simulink model "GNC_integrated"  (R2023a)
settings: Solver=VariableStepAuto  StartTime=0.0  StopTime=200  RelTol=1e-3
undefined symbols (not defined in the file or in its folder): param
libraries: eeGeneralControl x12, simulink_extras x6, uavalgslib x3, simulink x2, SignalEditorBlockLib x1, sharedTrackingLibrary x1
settings Model: Creator=timme  LastModifiedBy=jipva

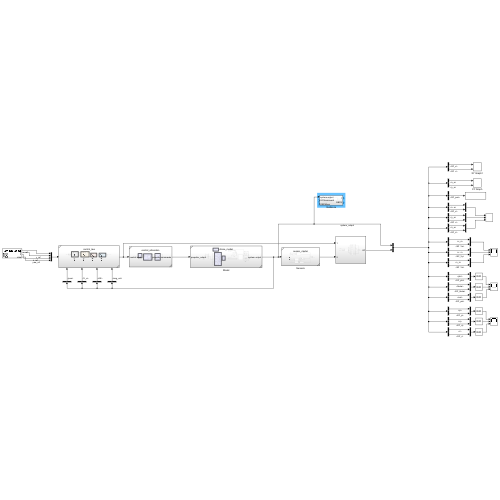
[thumbnail: Simulink's stored preview of the top-level diagram]
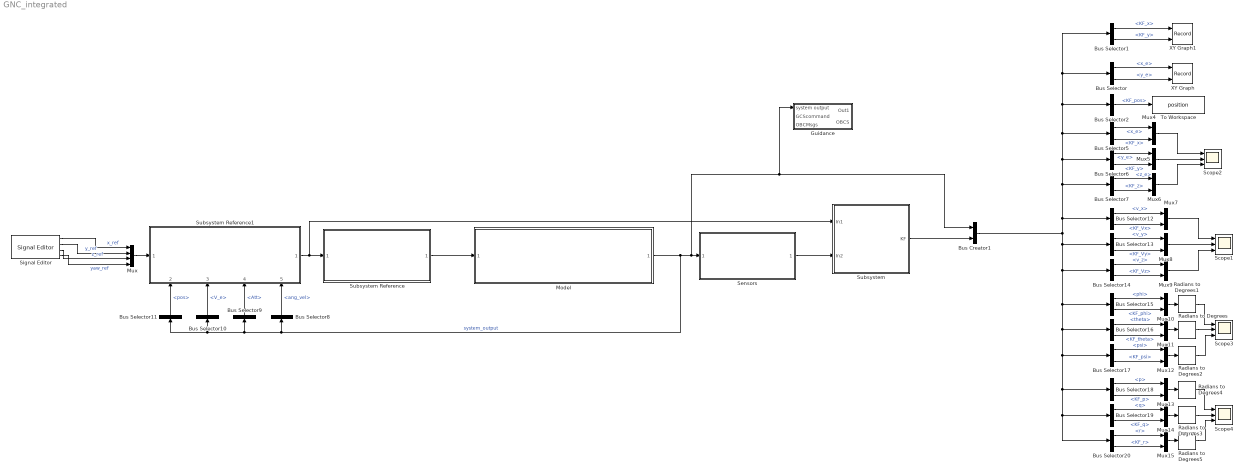
== system GNC_integrated ==
  Bus Creator1 : BusCreator  Inputs=2
  Bus Selector : BusSelector  OutputSignals=system_output.pos.x_e,system_output.pos.y_e
  Bus Selector1 : BusSelector  OutputSignals=KF.KF_pos.KF_x,KF.KF_pos.KF_y
  Bus Selector10 : BusSelector  OutputSignals=V_e
  Bus Selector11 : BusSelector  OutputSignals=pos
  Bus Selector12 : BusSelector  OutputSignals=system_output.V_e.v_x,KF.KF_vel.KF_Vx
  Bus Selector13 : BusSelector  OutputSignals=system_output.V_e.v_y,KF.KF_vel.KF_Vy
  Bus Selector14 : BusSelector  OutputSignals=system_output.V_e.v_z,KF.KF_vel.KF_Vz
  Bus Selector15 : BusSelector  OutputSignals=system_output.Att.phi,KF.KF_att.KF_phi
  Bus Selector16 : BusSelector  OutputSignals=system_output.Att.theta,KF.KF_att.KF_theta
  Bus Selector17 : BusSelector  OutputSignals=system_output.Att.psi,KF.KF_att.KF_psi
  Bus Selector18 : BusSelector  OutputSignals=system_output.ang_vel.p,KF.KF_omega.KF_p
  Bus Selector19 : BusSelector  OutputSignals=system_output.ang_vel.q,KF.KF_omega.KF_q
  Bus Selector2 : BusSelector  OutputSignals=KF.KF_pos
  Bus Selector20 : BusSelector  OutputSignals=system_output.ang_vel.r,KF.KF_omega.KF_r
  Bus Selector5 : BusSelector  OutputSignals=system_output.pos.x_e,KF.KF_pos.KF_x
  Bus Selector6 : BusSelector  OutputSignals=system_output.pos.y_e,KF.KF_pos.KF_y
  Bus Selector7 : BusSelector  OutputSignals=system_output.pos.z_e,KF.KF_pos.KF_z
  Bus Selector8 : BusSelector  OutputSignals=ang_vel
  Bus Selector9 : BusSelector  OutputSignals=Att
  Guidance : Subsystem
  Model : Subsystem  ReferencedSubsystem=drone_model
  Mux : Mux
  Mux{4..15} (12 alike) : Mux  Inputs=2
  Radians to Degrees{,1..5} (6 alike) : simulink_extras/Transformations/Radians to Degrees
  Scope{1..4} (4 alike) : Scope  NumInputPorts=3
  Sensors : Subsystem  ReferencedSubsystem=sensor_model
  Signal Editor : SignalEditorBlockLib/Signal Editor  FileName=C:\Users\jipva\MATLAB\Projects\drone\Detailed design phase\guidance\full_system_reference.mat  ActiveScenario=StandardScenario  ActiveSignal=yaw  IsBus=off  OutputBusObjectStr=Bus: BusObject  SampleTime=param.dt  ZeroCross=off  OutputAfterFinalValue=Setting to zero  Unit=inherit  PreserveSignalName=on  ApplySigPropsToAllScenarios=on
  Subsystem : Subsystem
  Subsystem Reference : Subsystem  ReferencedSubsystem=control_allocation
  Subsystem Reference1 : Subsystem  ReferencedSubsystem=control_law
      settings: PortSchema="{\"entries\":[{\"content\":{\"sides\":[{\"content\":{\"connectorIds\":[\"In1\"]},\"type\":\"ConnectorPlacement.EquallySpacedRectSide\",\"uuid\":\"cbb659e7-d19a-4e68-9ae7-e5e39426296b\"},{\"content\":{\"connectorIds\":[\"Out1\"],\"side\":\"RIGHT\"},\"type\":\"ConnectorPlacement.EquallySpacedRectSide\",\"uuid\":\"c9f08a4e-80d9-41bf-93e6-4cfd11b32426\"},{\"content\":{\"side\":\"TOP\"},\"type\":\"ConnectorPlacement.EquallySpacedRectSide\",\"uuid\":\"8eafc22d-128e-4ca7-9eba-2c3fd299252c\"},{\"content\":{\"connectorIds\":[\"In2\",\"In3\",\"In4\",\"In5\"],\"side\":\"BOTTOM\"},\"type\":\"ConnectorPlacement.EquallySpacedRectSide\",\"uuid\":\"abe1dc09-e6b8-433e-beaf-ba54ebcb4b47\"}]},\"type\":\"ConnectorPlacement.EquallySpacedConnector\",\"uuid\":\"085ffc95-65e8-4235-be8d-72c324b16b8b\"}],\"packageUris\":[\"http://schema.mathworks.com/mf0/Connector/R2020b\"],\"version\":\"1.0\"}"
  To Workspace : ToWorkspace  VariableName=position  SaveFormat=Timeseries  SampleTime=param.dt
  XY Graph : Record  FileSettingsInternal="{\"entries\":[{\"content\":{\"excelSettings\":{\"content\":{},\"type\":\"Streamout.ExcelSettings\"}},\"type\":\"Streamout.FileSettingStorage\",\"uuid\":\"\"}],\"packageUris\":[\"http:\\/\\/schema.mathworks.com\\/mf0\\/streamout_blocks\\/R2020a\"],\"version\":\"1.0\"}"  Layout=[1 1]  SignalsInternal="{\"entries\":[{\"content\":{\"signals\":[{\"content\":{\"blockPath\":[],\"dimensions\":[1],\"domain\":\"\",\"lineColor\":\"#a2142f\",\"plots\":[1],\"port\":1,\"signalID\":34,\"signalName\":\"<x_e>\"},\"type\":\"RecordBlkView.Signal\",\"uuid\":\"\"},{\"content\":{\"blockPath\":[],\"dimensions\":[1],\"domain\":\"\",\"lineColor\":\"#139fff\",\"plots\":[1],\"port\":2,\"signalID\":37,\"signalName\":\"<y_e>\"},\"type\":\"RecordBlkView.Signal\",\"uuid\":\"\"}]},\"type\":\"RecordBlkView.InputSignals\",\"uuid\":\"\"}],\"packageUris\":[\"http:\\/\\/schema.mathworks.com\\/mf0\\/streamout_blocks\\/R2020a\"],\"version\":\"1.0\"}"  VisualizationBindings="{\"xyplotplugin\":{\"info\":[{\"series\":[{\"bindingParametersList\":[{\"parameter\":\"X-Axis\",\"signalID\":34,\"signalName\":\"<x_e>\"},{\"parameter\":\"Y-Axis\",\"signalID\":37,\"signalName\":\"<y_e>\"}],\"seriesID\":47186}],\"subplotID\":1}]}}"  CompatibilityTag=XY
  XY Graph1 : Record  FileSettingsInternal="{\"entries\":[{\"content\":{\"excelSettings\":{\"content\":{},\"type\":\"Streamout.ExcelSettings\"}},\"type\":\"Streamout.FileSettingStorage\",\"uuid\":\"\"}],\"packageUris\":[\"http:\\/\\/schema.mathworks.com\\/mf0\\/streamout_blocks\\/R2020a\"],\"version\":\"1.0\"}"  Layout=[1 1]  SignalsInternal="{\"entries\":[{\"content\":{\"signals\":[{\"content\":{\"blockPath\":[],\"dimensions\":[1],\"domain\":\"\",\"lineColor\":\"#a2142f\",\"plots\":[1],\"port\":1,\"signalID\":26,\"signalName\":\"Second-Order Filter3\"},\"type\":\"RecordBlkView.Signal\",\"uuid\":\"\"},{\"content\":{\"blockPath\":[],\"dimensions\":[1],\"domain\":\"\",\"lineColor\":\"#139fff\",\"plots\":[1],\"port\":2,\"signalID\":29,\"signalName\":\"Second-Order Filter4\"},\"type\":\"RecordBlkView.Signal\",\"uuid\":\"\"}]},\"type\":\"RecordBlkView.InputSignals\",\"uuid\":\"\"}],\"packageUris\":[\"http:\\/\\/schema.mathworks.com\\/mf0\\/streamout_blocks\\/R2020a\"],\"version\":\"1.0\"}"  VisualizationBindings="{\"xyplotplugin\":{\"info\":[{\"series\":[{\"bindingParametersList\":[{\"parameter\":\"X-Axis\",\"signalID\":26,\"signalName\":\"Second-Order Filter3\"},{\"parameter\":\"Y-Axis\",\"signalID\":29,\"signalName\":\"Second-Order Filter4\"}],\"seriesID\":35333}],\"subplotID\":1}]}}"  CompatibilityTag=XY
  wires:
  Model/1 -> Guidance/1(system output), Bus Creator1/1, Sensors/1, Bus Selector11/1, Bus Selector10/1, Bus Selector9/1, Bus Selector8/1  "system_output"
  Subsystem Reference1/1 -> Subsystem/1(In1), Subsystem Reference/1
  Bus Selector5/1 -> Mux4/1  "<x_e>"
  Bus Selector5/2 -> Mux4/2  "<KF_x>"
  Bus Selector6/1 -> Mux5/1  "<y_e>"
  Bus Selector6/2 -> Mux5/2  "<KF_y>"
  Bus Selector7/2 -> Mux6/2  "<KF_z>"
  Bus Selector7/1 -> Mux6/1  "<z_e>"
  Bus Selector8/1 -> Subsystem Reference1/5  "<ang_vel>"
  Bus Selector9/1 -> Subsystem Reference1/4  "<Att>"
  Bus Selector10/1 -> Subsystem Reference1/3  "<V_e>"
  Bus Selector11/1 -> Subsystem Reference1/2  "<pos>"
  Bus Selector12/2 -> Mux7/2  "<KF_Vx>"
  Bus Selector12/1 -> Mux7/1  "<v_x>"
  Bus Selector13/1 -> Mux8/1  "<v_y>"
  Bus Selector14/2 -> Mux9/2  "<KF_Vz>"
  Bus Selector14/1 -> Mux9/1  "<v_z>"
  Bus Selector13/2 -> Mux8/2  "<KF_Vy>"
  Bus Selector16/2 -> Mux11/2  "<KF_theta>"
  Mux12/1 -> Radians to Degrees2/1
  Mux11/1 -> Radians to Degrees/1
  Bus Selector17/2 -> Mux12/2  "<KF_psi>"
  Bus Selector17/1 -> Mux12/1  "<psi>"
  Bus Selector15/2 -> Mux10/2  "<KF_phi>"
  Mux10/1 -> Radians to Degrees1/1
  Bus Selector15/1 -> Mux10/1  "<phi>"
  Bus Selector16/1 -> Mux11/1  "<theta>"
  Bus Selector19/2 -> Mux14/2  "<KF_q>"
  Bus Selector18/2 -> Mux13/2  "<KF_p>"
  Mux13/1 -> Radians to Degrees4/1
  Bus Selector20/1 -> Mux15/1  "<r>"
  Bus Selector18/1 -> Mux13/1  "<p>"
  Mux15/1 -> Radians to Degrees5/1
  Bus Selector20/2 -> Mux15/2  "<KF_r>"
  Mux14/1 -> Radians to Degrees3/1
  Bus Selector19/1 -> Mux14/1  "<q>"
  Signal Editor/2 -> Mux/2  "y_ref"
  Signal Editor/1 -> Mux/1  "x_ref"
  Signal Editor/3 -> Mux/3  "z_ref"
  Signal Editor/4 -> Mux/4  "yaw_ref"
  Mux/1 -> Subsystem Reference1/1
  Subsystem Reference/1 -> Model/1
  Bus Selector/1 -> XY Graph/1  "<x_e>"
  Bus Selector/2 -> XY Graph/2  "<y_e>"
  Bus Creator1/1 -> Bus Selector13/1, Bus Selector14/1, Bus Selector20/1, Bus Selector19/1, Bus Selector18/1, Bus Selector17/1, Bus Selector16/1, Bus Selector15/1, Bus Selector12/1, Bus Selector7/1, Bus Selector6/1, Bus Selector2/1, Bus Selector1/1, Bus Selector/1, Bus Selector5/1
  Mux5/1 -> Scope2/2
  Mux4/1 -> Scope2/1
  Mux6/1 -> Scope2/3
  Mux8/1 -> Scope1/2
  Mux9/1 -> Scope1/3
  Mux7/1 -> Scope1/1
  Radians to Degrees2/1 -> Scope3/3
  Radians to Degrees1/1 -> Scope3/1
  Radians to Degrees/1 -> Scope3/2
  Radians to Degrees5/1 -> Scope4/3
  Radians to Degrees4/1 -> Scope4/1
  Radians to Degrees3/1 -> Scope4/2
  Bus Selector1/1 -> XY Graph1/1  "<KF_x>"
  Bus Selector1/2 -> XY Graph1/2  "<KF_y>"
  Sensors/1 -> Subsystem/2(In2)
  Subsystem/1(KF) -> Bus Creator1/2
  Bus Selector2/1 -> To Workspace/1  "<KF_pos>"

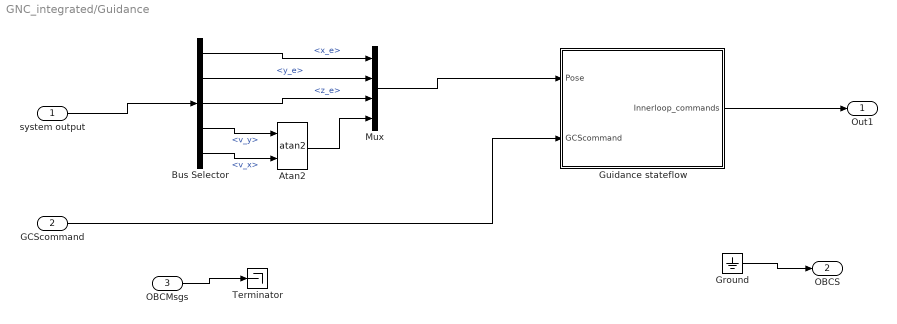
== system GNC_integrated/Guidance ==
  system output : Inport
  GCScommand : Inport  Port=2
  OBCMsgs : Inport  Port=3
  Atan2 : Trigonometry  Operator=atan2
  Bus Selector : BusSelector  OutputSignals=pos.x_e,pos.y_e,pos.z_e,V_e.v_y,V_e.v_x
  Ground : Ground
  Guidance stateflow : Subsystem
  Mux : Mux
  Terminator : Terminator
  Out1 : Outport
  OBCS : Outport  Port=2
  wires:
  system output/1 -> Bus Selector/1
  Bus Selector/4 -> Atan2/1  "<v_y>"
  Bus Selector/5 -> Atan2/2  "<v_x>"
  Bus Selector/3 -> Mux/3  "<z_e>"
  Bus Selector/2 -> Mux/2  "<y_e>"
  Bus Selector/1 -> Mux/1  "<x_e>"
  Atan2/1 -> Mux/4
  Mux/1 -> Guidance stateflow/1(Pose)
  GCScommand/1 -> Guidance stateflow/2(GCScommand)
  OBCMsgs/1 -> Terminator/1
  Guidance stateflow/1(Innerloop_commands) -> Out1/1
  Ground/1 -> OBCS/1

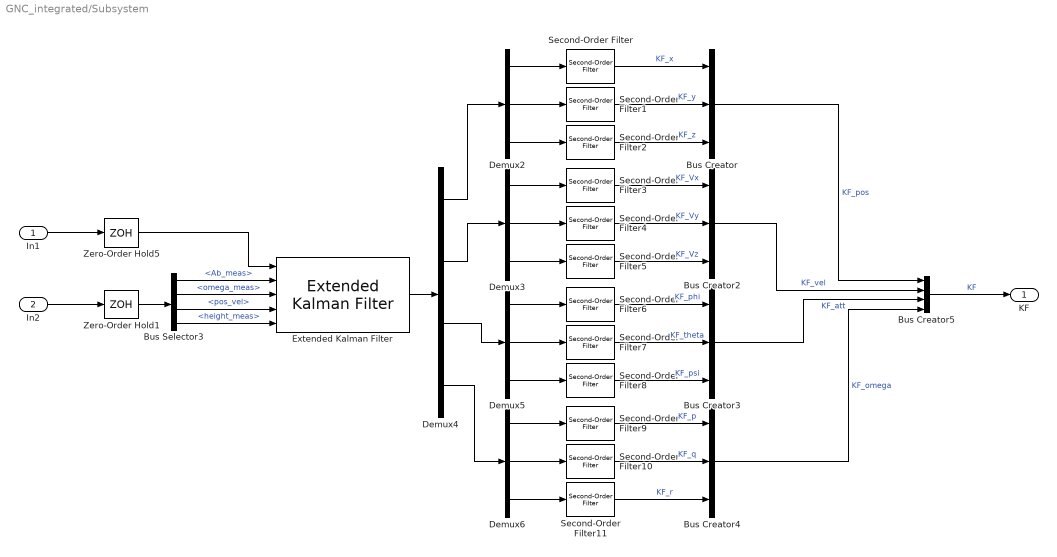
== system GNC_integrated/Subsystem ==
  In1 : Inport
  In2 : Inport  Port=2
  Bus Creator{,2..4} (4 alike) : BusCreator  Inputs=3
  Bus Creator5 : BusCreator  Inputs=4
  Bus Selector3 : BusSelector  OutputSignals=Ab_meas,omega_meas,pos_vel,height_meas
  Demux{2..3,5..6} (4 alike) : Demux  Outputs=3
  Demux4 : Demux
  Extended Kalman Filter : sharedTrackingLibrary/Extended Kalman Filter  StateTransitionFcn=stateTransition  HasStateTransitionJacobianFcn=off  HasAdditiveProcessNoise=Additive  ProcessNoise=10  HasTimeVaryingProcessNoise=off  HasStateTransitionFcnExtraArgument=1  InitialState=zeros(12,1)  InitialStateCovariance=zeros(12)  MeasurementFcn1=accelerometer_model  HasMeasurementJacobianFcn1=off  HasMeasurementEnablePort1=off  HasAdditiveMeasurementNoise1=Additive  MeasurementNoise1=diag([100 100 100])  HasTimeVaryingMeasurementNoise1=off  HasMeasurementFcnExtraArgument1=0  HasMeasurementWrapping1=off  MeasurementFcn2=gyrometer_model  HasMeasurementJacobianFcn2=off  HasMeasurementEnablePort2=off  HasAdditiveMeasurementNoise2=Additive  MeasurementNoise2=eye(3)  HasTimeVaryingMeasurementNoise2=off  HasMeasurementFcnExtraArgument2=0  HasMeasurementWrapping2=off  MeasurementFcn3=GPS_model  HasMeasurementJacobianFcn3=off  HasMeasurementEnablePort3=off  HasAdditiveMeasurementNoise3=Additive  MeasurementNoise3=diag([10 10 100 0.1 0.1 0.1])  HasTimeVaryingMeasurementNoise3=off  HasMeasurementFcnExtraArgument3=0  HasMeasurementWrapping3=off  MeasurementFcn4=Barometer_model  HasMeasurementJacobianFcn4=off  HasMeasurementEnablePort4=off  HasAdditiveMeasurementNoise4=Additive  MeasurementNoise4=0.01  HasTimeVaryingMeasurementNoise4=off  HasMeasurementFcnExtraArgument4=0  HasMeasurementWrapping4=off  MeasurementFcn5=myMeasurementFcn  HasMeasurementJacobianFcn5=off  HasMeasurementEnablePort5=off  HasAdditiveMeasurementNoise5=Additive  MeasurementNoise5=1  HasTimeVaryingMeasurementNoise5=off  HasMeasurementFcnExtraArgument5=0  HasMeasurementWrapping5=off  EnableMultirate=off  StateTransitionFcnSampleTime=1  MeasurementFcn1SampleTime=1  MeasurementFcn2SampleTime=1  MeasurementFcn3SampleTime=1  MeasurementFcn4SampleTime=1  MeasurementFcn5SampleTime=1  UseCurrentEstimator=on  OutputStateCovariance=off  DataType=double  SampleTime=0.01  NumberOfMeasurements=4
  Second-Order Filter{,1..11} (12 alike) : eeGeneralControl/Second-Order Filter  FilterType=Low-pass  fn=10  Zeta=0.707  Ts=param.dt  A0=0  Ph0=0  f0=0  b0=0
      settings: LibrarySourceBlock=ee_sl_lib/General Control/Second-Order Filter
  Zero-Order Hold1 : ZeroOrderHold  SampleTime=param.dt
  Zero-Order Hold5 : ZeroOrderHold  SampleTime=param.dt
  KF : Outport
  wires:
  Demux5/2 -> Second-Order Filter7/1
  Bus Selector3/2 -> Extended Kalman Filter/3  "<omega_meas>"
  Demux6/1 -> Second-Order Filter9/1
  Bus Selector3/3 -> Extended Kalman Filter/4  "<pos_vel>"
  Demux2/3 -> Second-Order Filter2/1
  Zero-Order Hold5/1 -> Extended Kalman Filter/1
  Demux3/1 -> Second-Order Filter3/1
  Zero-Order Hold1/1 -> Bus Selector3/1
  Demux6/2 -> Second-Order Filter10/1
  Demux6/3 -> Second-Order Filter11/1
  Demux5/3 -> Second-Order Filter8/1
  Bus Creator2/1 -> Bus Creator5/2  "KF_vel"
  Bus Creator/1 -> Bus Creator5/1  "KF_pos"
  Demux4/2 -> Demux3/1
  Demux3/3 -> Second-Order Filter5/1
  Demux2/1 -> Second-Order Filter/1
  Bus Creator4/1 -> Bus Creator5/4  "KF_omega"
  Demux4/1 -> Demux2/1
  Demux5/1 -> Second-Order Filter6/1
  Bus Selector3/1 -> Extended Kalman Filter/2  "<Ab_meas>"
  Demux3/2 -> Second-Order Filter4/1
  Bus Selector3/4 -> Extended Kalman Filter/5  "<height_meas>"
  Bus Creator3/1 -> Bus Creator5/3  "KF_att"
  Demux4/4 -> Demux6/1
  In2/1 -> Zero-Order Hold1/1
  Second-Order Filter1/1 -> Bus Creator/2  "KF_y"
  Extended Kalman Filter/1 -> Demux4/1
  Demux4/3 -> Demux5/1
  Bus Creator5/1 -> KF/1  "KF"
  In1/1 -> Zero-Order Hold5/1
  Second-Order Filter/1 -> Bus Creator/1  "KF_x"
  Demux2/2 -> Second-Order Filter1/1
  Second-Order Filter2/1 -> Bus Creator/3  "KF_z"
  Second-Order Filter3/1 -> Bus Creator2/1  "KF_Vx"
  Second-Order Filter4/1 -> Bus Creator2/2  "KF_Vy"
  Second-Order Filter5/1 -> Bus Creator2/3  "KF_Vz"
  Second-Order Filter6/1 -> Bus Creator3/1  "KF_phi"
  Second-Order Filter7/1 -> Bus Creator3/2  "KF_theta"
  Second-Order Filter8/1 -> Bus Creator3/3  "KF_psi"
  Second-Order Filter9/1 -> Bus Creator4/1  "KF_p"
  Second-Order Filter10/1 -> Bus Creator4/2  "KF_q"
  Second-Order Filter11/1 -> Bus Creator4/3  "KF_r"

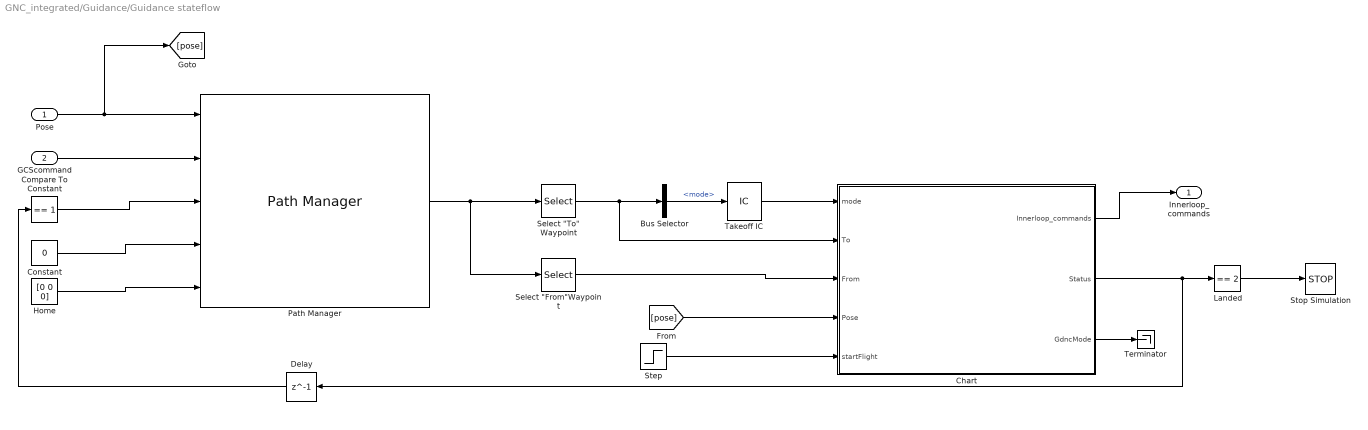
== system GNC_integrated/Guidance/Guidance stateflow ==
  Pose : Inport
  GCScommand : Inport  Port=2
  Bus Selector : BusSelector  OutputSignals=mode
  Chart : Stateflow chart  TreatAsAtomicUnit=on
      settings: PortSchema="{\"entries\":[{\"content\":{\"sides\":[{\"content\":{\"connectorIds\":[\"In1\",\"In3\",\"In4\",\"In2\",\"In5\"]},\"type\":\"ConnectorPlacement.EquallySpacedRectSide\",\"uuid\":\"d234d877-22d9-4518-b5ba-a604db0bf90b\"},{\"content\":{\"connectorIds\":[\"Out1\",\"Out2\",\"Out3\"],\"side\":\"RIGHT\"},\"type\":\"ConnectorPlacement.EquallySpacedRectSide\",\"uuid\":\"0dfe34a8-7c44-4a97-9042-ef916a7aa529\"},{\"content\":{\"side\":\"TOP\"},\"type\":\"ConnectorPlacement.EquallySpacedRectSide\",\"uuid\":\"69e1da7c-b0a2-43d5-a7f5-1531e368ea9d\"}]},\"type\":\"ConnectorPlacement.EquallySpacedConnector\",\"uuid\":\"b60a6dee-5aca-438c-8d1f-1665cdae5849\"}],\"packageUris\":[\"http://schema.mathworks.com/mf0/Connector/R2020b\"],\"version\":\"1.0\"}"
  Compare To Constant : simulink/Logic and Bit Operations/Compare To Constant  relop===  const=1  OutDataTypeStr=boolean
  Constant : Constant  Value=0
  Delay : Delay  DelayLength=1  InitialCondition=0
  Home : Constant  Value=[0 0 0]
  Landed : simulink/Logic and Bit Operations/Compare To Constant  relop===  const=2  OutDataTypeStr=boolean
  Path Manager : uavalgslib/Path Manager  UAVType=multirotor  LoiterRadius=25  dataType=double  inputBusName='UAVPathManagerBus'  SimulateUsing=Interpreted execution
  "Select \"From\"Waypoint" : Selector  InputPortWidth=2  IndexOptions=Index vector (dialog)  Indices=2  OutputSizes=1
  "Select \"To\" Waypoint" : Selector  InputPortWidth=2  IndexOptions=Index vector (dialog)  Indices=1  OutputSizes=1
  Step : Step  Time=0.5  SampleTime=0.02
  Stop Simulation : Stop
  Takeoff IC : InitialCondition
  Terminator : Terminator
  Innerloop_commands : Outport
  wires:
  Pose/1 -> [pose], Path Manager/1
  GCScommand/1 -> Path Manager/2
  Home/1 -> Path Manager/5
  Constant/1 -> Path Manager/4
  Path Manager/1 -> "Select \"From\"Waypoint"/1, "Select \"To\" Waypoint"/1
  "Select \"To\" Waypoint"/1 -> Chart/3(To), Bus Selector/1
  Bus Selector/1 -> Takeoff IC/1  "<mode>"
  "Select \"From\"Waypoint"/1 -> Chart/4(From)
  Delay/1 -> Compare To Constant/1
  Compare To Constant/1 -> Path Manager/3
  [pose] -> Chart/2(Pose)
  Chart/1(Innerloop_commands) -> Innerloop_commands/1
  Takeoff IC/1 -> Chart/1(mode)
  Step/1 -> Chart/5(startFlight)
  Chart/3(GdncMode) -> Terminator/1
  Chart/2(Status) -> Delay/1, Landed/1
  Landed/1 -> Stop Simulation/1

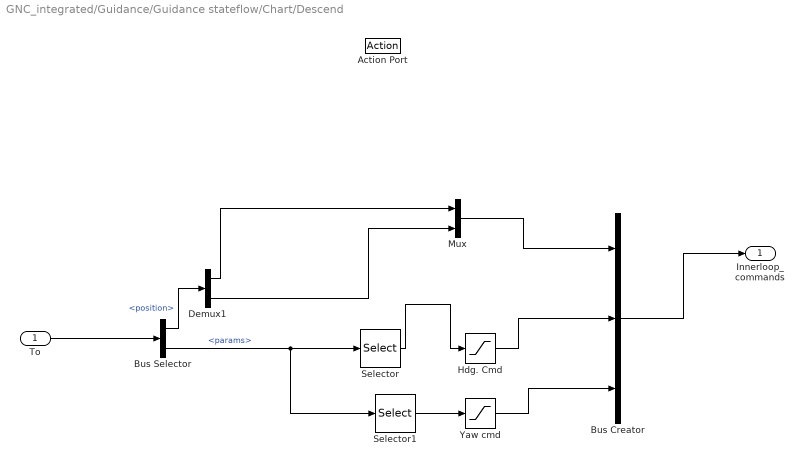
== system GNC_integrated/Guidance/Guidance stateflow/Chart/Descend ==
  To : Inport
  Action Port : ActionPort
      settings: CopyFcn=Stateflow.SLINSF.SimulinkMan.removeBlockPreDeleteFcn  PreDeleteFcn=Stateflow.SLINSF.SimulinkMan.unsafePredeleteFcn
  Bus Creator : BusCreator  Inputs=3
  Bus Selector : BusSelector  OutputSignals=position,params
  Demux1 : Demux  Outputs=2
  Hdg. Cmd : Saturate
  Mux : Mux  Inputs=2
  Selector : Selector  InputPortWidth=4  IndexOptions=Index vector (dialog)  Indices=4  OutputSizes=1
  Selector1 : Selector  InputPortWidth=4  IndexOptions=Index vector (dialog)  Indices=4  OutputSizes=1
  Yaw cmd : Saturate  UpperLimit=pi  LowerLimit=-pi
  Innerloop_commands : Outport
  wires:
  Bus Selector/1 -> Demux1/1  "<position>"
  Demux1/2 -> Mux/2
  Mux/1 -> Bus Creator/1
  Bus Selector/2 -> Selector1/1, Selector/1  "<params>"
  Selector1/1 -> Yaw cmd/1
  Demux1/1 -> Mux/1
  Hdg. Cmd/1 -> Bus Creator/2
  Selector/1 -> Hdg. Cmd/1
  Yaw cmd/1 -> Bus Creator/3
  Bus Creator/1 -> Innerloop_commands/1
  To/1 -> Bus Selector/1

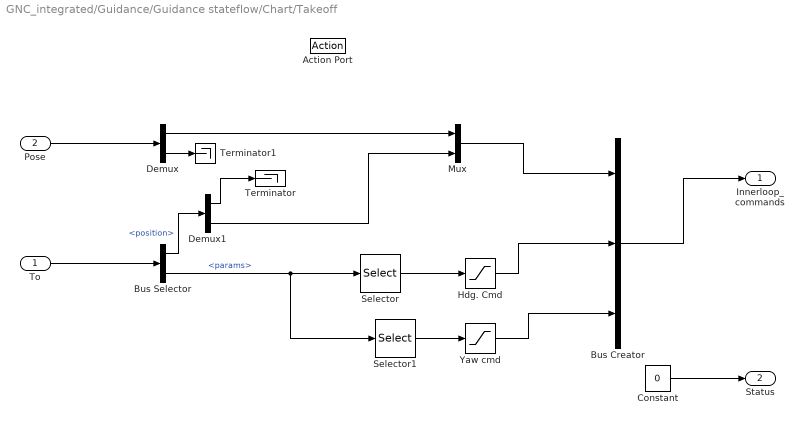
== system GNC_integrated/Guidance/Guidance stateflow/Chart/Takeoff ==
  To : Inport
  Pose : Inport  Port=2
  Action Port : ActionPort
      settings: CopyFcn=Stateflow.SLINSF.SimulinkMan.removeBlockPreDeleteFcn  PreDeleteFcn=Stateflow.SLINSF.SimulinkMan.unsafePredeleteFcn
  Bus Creator : BusCreator  Inputs=3
  Bus Selector : BusSelector  OutputSignals=position,params
  Constant : Constant  Value=0
  Demux : Demux  Outputs=2
  Demux1 : Demux  Outputs=2
  Hdg. Cmd : Saturate
  Mux : Mux  Inputs=2
  Selector : Selector  InputPortWidth=4  IndexOptions=Index vector (dialog)  Indices=4  OutputSizes=1
  Selector1 : Selector  InputPortWidth=4  IndexOptions=Index vector (dialog)  Indices=4  OutputSizes=1
  Terminator : Terminator
  Terminator1 : Terminator
  Yaw cmd : Saturate  UpperLimit=pi  LowerLimit=-pi
  Innerloop_commands : Outport
  Status : Outport  Port=2
  wires:
  Pose/1 -> Demux/1
  Demux/1 -> Mux/1
  Mux/1 -> Bus Creator/1
  To/1 -> Bus Selector/1
  Bus Selector/1 -> Demux1/1  "<position>"
  Demux1/1 -> Terminator/1
  Demux1/2 -> Mux/2
  Bus Selector/2 -> Selector1/1, Selector/1  "<params>"
  Bus Creator/1 -> Innerloop_commands/1
  Demux/2 -> Terminator1/1
  Hdg. Cmd/1 -> Bus Creator/2
  Selector1/1 -> Yaw cmd/1
  Selector/1 -> Hdg. Cmd/1
  Yaw cmd/1 -> Bus Creator/3
  Constant/1 -> Status/1

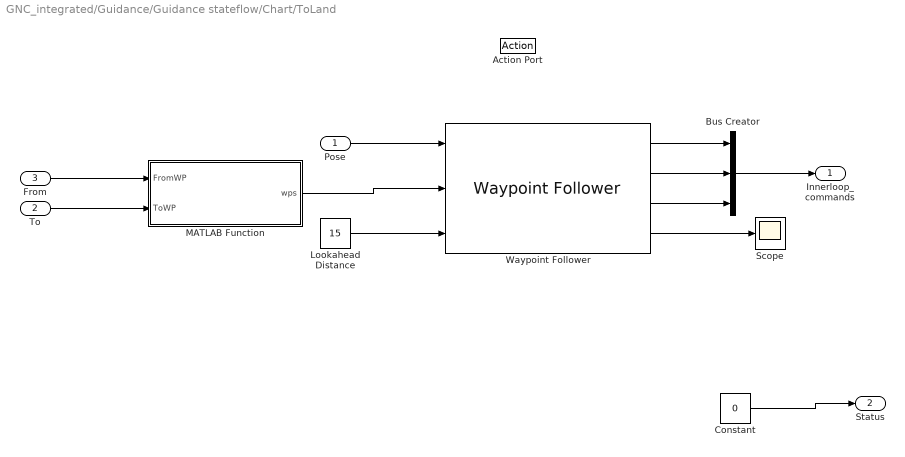
== system GNC_integrated/Guidance/Guidance stateflow/Chart/ToLand ==
  Pose : Inport
  To : Inport  Port=2
  From : Inport  Port=3
  Action Port : ActionPort
      settings: CopyFcn=Stateflow.SLINSF.SimulinkMan.removeBlockPreDeleteFcn  PreDeleteFcn=Stateflow.SLINSF.SimulinkMan.unsafePredeleteFcn
  Bus Creator : BusCreator  Inputs=3
  Constant : Constant  Value=0
  Lookahead Distance : Constant  Value=15
  MATLAB Function : MATLAB Function  TreatAsAtomicUnit=on
  Scope : Scope
  Waypoint Follower : uavalgslib/Waypoint Follower  UAVType=multirotor  StartFrom=first  TransitionRadiusSource=internal  TransitionRadius=10  MinLookaheadDistance=0.1  YawInput=off  ShowCrossTrackErrorOutput=off  ShowStatusOutput=off  SimulateUsing=Interpreted execution
  Innerloop_commands : Outport
  Status : Outport  Port=2
  wires:
  To/1 -> MATLAB Function/2(ToWP)
  MATLAB Function/1(wps) -> Waypoint Follower/2
  Waypoint Follower/1 -> Bus Creator/1
  Bus Creator/1 -> Innerloop_commands/1
  From/1 -> MATLAB Function/1(FromWP)
  Pose/1 -> Waypoint Follower/1
  Waypoint Follower/2 -> Bus Creator/2
  Waypoint Follower/4 -> Scope/1
  Lookahead Distance/1 -> Waypoint Follower/3
  Waypoint Follower/3 -> Bus Creator/3
  Constant/1 -> Status/1

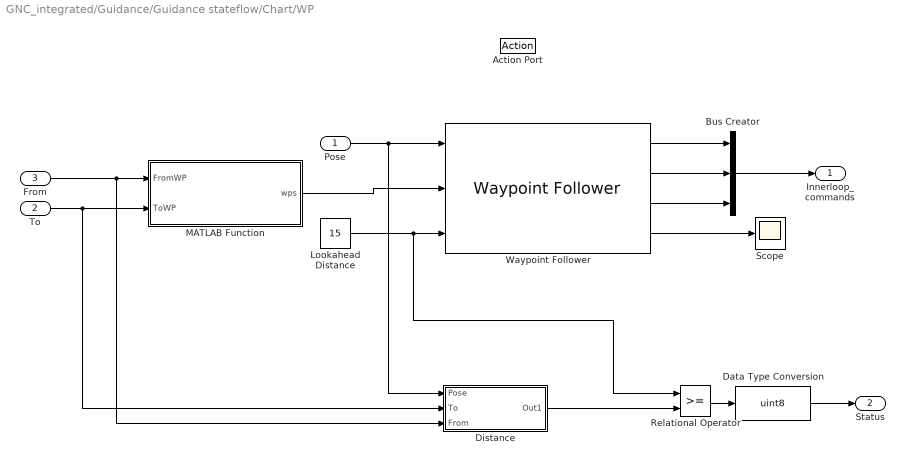
== system GNC_integrated/Guidance/Guidance stateflow/Chart/WP ==
  Pose : Inport
  To : Inport  Port=2
  From : Inport  Port=3
  Action Port : ActionPort
      settings: CopyFcn=Stateflow.SLINSF.SimulinkMan.removeBlockPreDeleteFcn  PreDeleteFcn=Stateflow.SLINSF.SimulinkMan.unsafePredeleteFcn
  Bus Creator : BusCreator  Inputs=3
  Data Type Conversion : DataTypeConversion  OutDataTypeStr=uint8  SaturateOnIntegerOverflow=off  RndMeth=Floor
  Distance : Subsystem
  Lookahead Distance : Constant  Value=15
  MATLAB Function : MATLAB Function  TreatAsAtomicUnit=on
  Relational Operator : RelationalOperator  OutDataTypeStr=boolean  RndMeth=Simplest  InputSameDT=off
  Scope : Scope
  Waypoint Follower : uavalgslib/Waypoint Follower  UAVType=multirotor  StartFrom=first  TransitionRadiusSource=internal  TransitionRadius=10  MinLookaheadDistance=0.1  YawInput=off  ShowCrossTrackErrorOutput=off  ShowStatusOutput=off  SimulateUsing=Interpreted execution
  Innerloop_commands : Outport
  Status : Outport  Port=2
  wires:
  To/1 -> Distance/2(To), MATLAB Function/2(ToWP)
  MATLAB Function/1(wps) -> Waypoint Follower/2
  Waypoint Follower/1 -> Bus Creator/1
  Data Type Conversion/1 -> Status/1
  Bus Creator/1 -> Innerloop_commands/1
  From/1 -> Distance/3(From), MATLAB Function/1(FromWP)
  Pose/1 -> Distance/1(Pose), Waypoint Follower/1
  Waypoint Follower/2 -> Bus Creator/2
  Waypoint Follower/4 -> Scope/1
  Relational Operator/1 -> Data Type Conversion/1
  Distance/1(Out1) -> Relational Operator/2
  Lookahead Distance/1 -> Relational Operator/1, Waypoint Follower/3
  Waypoint Follower/3 -> Bus Creator/3

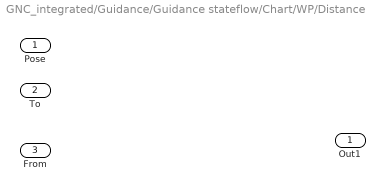
== system GNC_integrated/Guidance/Guidance stateflow/Chart/WP/Distance ==
  Pose : Inport
  To : Inport  Port=2
  From : Inport  Port=3
  Out1 : Outport

== matlab function GNC_integrated/Guidance/Guidance stateflow/Chart/ToLand/MATLAB Function ==
  data: FromWP input; wps output; ToWP input
function wps = getLandingWaypoint(FromWP, ToWP)

persistent outWPS

if isempty(outWPS)
    outWPS = single(zeros(2,4));
end

outWPS(1,:) = [FromWP.position' FromWP.params(4)];
outWPS(2,:) = [ToWP.position(1:2)' FromWP.position(3) ToWP.params(4)];

wps = outWPS;

== stateflow chart GNC_integrated/Guidance/Guidance stateflow/Chart ==
  state Guidance logic
  state Onground
  state Takeoff
  state WP
  state Name
  state ToLand
  state Descend
  (default) -> Guidance logic [order 1]
  (default) -> Onground [order 2]
  Onground -> (junction 12) : [startFlight == 1]
  Guidance logic -> (junction 12) : [hasChanged(mode)]
  (junction 12) -> Takeoff [order 1] : [mode == 1]
  Takeoff -> WP : [Pose(3) <=ToWP.postion(3)]{Status =1;}
  (junction 12) -> (junction 17) [order 2]
  (junction 17) -> WP [order 1] : [mode == 2]
  (junction 17) -> (junction 39) [order 2]
  (default) -> ToLand [order 3]
  (junction 39) -> Name
  Name -> Guidance logic : [Pose(3)>=-0.1]{Status=2;}
  ToLand -> Descend
  data: sf_internal_action_state_placeholder_data local double size=1 =0; sf_internal_action_state_placeholder_data local double size=1 =0; sf_internal_action_state_placeholder_data local double size=1 =0; sf_internal_action_state_placeholder_data local double size=1 =0; Innerloop_commands output; mode input; Pose input; To input; From input; startFlight input; Status output; GdncMode output

== matlab function GNC_integrated/Guidance/Guidance stateflow/Chart/WP/MATLAB Function ==
  data: FromWP input; wps output; ToWP input
function wps = getWaypointMission(FromWP, ToWP)

persistent outWPS

if isempty(outWPS)
    outWPS = single(zeros(2,4));
end

outWPS(1,:) = [FromWP.position' FromWP.params(4)];
outWPS(2,:) = [ToWP.position' ToWP.params(4)];

% for ii=1:2
%     outWPS(ii,1:3) = GCSMission(ii).position';
%     outWPS(ii,4) = GCSMission(ii).params(4);
% end

wps = outWPS;
